simulink model "SynRM_Model_field"  (Simulink 7.9)
settings: Solver=ode3  StartTime=0.0  StopTime=1  FixedStep=.00001  RelTol=1e-3
undefined symbols (not defined in the file): I_s_max, J, K_iid, K_iiq, K_ipd, K_ipq, K_wd, K_wi, K_wp, L_d, L_q, P_r, r_s, Ts_id, Ts_iq, U_max
libraries: simulink x7, simulink_extras x1
settings Model: Creator=KHANSED  LastModifiedBy=KHANSED

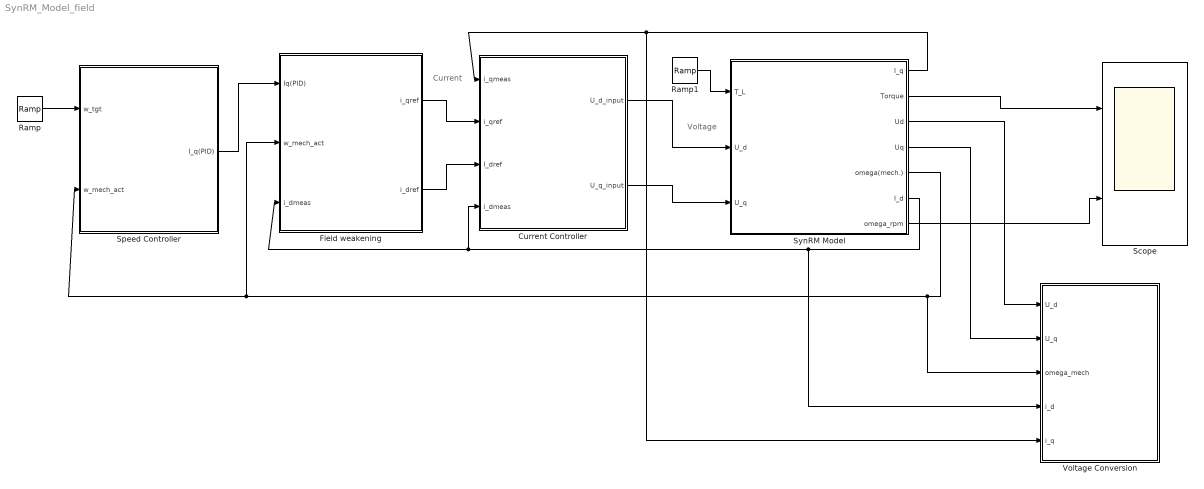
== system SynRM_Model_field ==
  note: Voltage
  note: Current
  Current Controller : Subsystem
  Field weakening : Subsystem
  Ramp : simulink/Sources/Ramp  slope=1500  start=0  X0=0
  Ramp1 : simulink/Sources/Ramp  slope=0  start=0.2  X0=0
  Scope : Scope  NumInputPorts=2
      settings: TimeRange=1  YMin=-0.012~-90.75  YMax=0.001~-89.7
  Speed Controller : Subsystem
  SynRM Model : Subsystem
  Voltage Conversion : Subsystem
  wires:
  SynRM Model/1(I_q) -> Current Controller/1(i_qmeas), Voltage Conversion/5(i_q)
  SynRM Model/6(I_d) -> Current Controller/4(i_dmeas), Field weakening/3(i_dmeas), Voltage Conversion/4(i_d)
  SynRM Model/5(omega(mech.)) -> Speed Controller/2(w_mech_act), Field weakening/2(w_mech_act), Voltage Conversion/3(omega_mech)
  Current Controller/1(U_d_input) -> SynRM Model/2(U_d)
  Current Controller/2(U_q_input) -> SynRM Model/3(U_q)
  SynRM Model/3(Ud) -> Voltage Conversion/1(U_d)
  SynRM Model/4(Uq) -> Voltage Conversion/2(U_q)
  SynRM Model/7(omega_rpm) -> Scope/2
  SynRM Model/2(Torque) -> Scope/1
  Ramp1/1 -> SynRM Model/1(T_L)
  Speed Controller/1(I_q(PID)) -> Field weakening/1(Iq(PID))
  Field weakening/2(i_dref) -> Current Controller/3(I_dref)
  Field weakening/1(i_qref) -> Current Controller/2(i_qref)
  Ramp/1 -> Speed Controller/1(w_tgt)

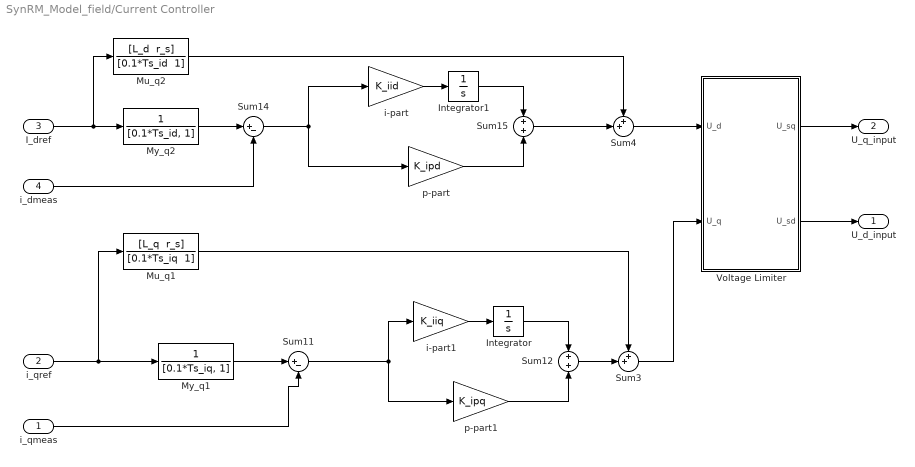
== system SynRM_Model_field/Current Controller ==
  i_qmeas : Inport
  i_qref : Inport  Port=2
  I_dref : Inport  Port=3
  i_dmeas : Inport  Port=4
  Integrator : Integrator
  Integrator1 : Integrator
  Mu_q1 : TransferFcn  Numerator="[L_q  r_s]"  Denominator="[0.1*Ts_iq  1]"
  Mu_q2 : TransferFcn  Numerator="[L_d  r_s]"  Denominator="[0.1*Ts_id  1]"
  My_q1 : TransferFcn  Denominator=[0.1*Ts_iq, 1]
  My_q2 : TransferFcn  Denominator=[0.1*Ts_id, 1]
  Sum11 : Sum  Inputs=|+-
  Sum12 : Sum
  Sum14 : Sum  Inputs=|+-
  Sum15 : Sum
  Sum3 : Sum  Inputs=++|
  Sum4 : Sum  Inputs=++|
  Voltage Limiter : Subsystem
  i-part : Gain  Gain=K_iid
  i-part1 : Gain  Gain=K_iiq
  p-part : Gain  Gain=K_ipd
  p-part1 : Gain  Gain=K_ipq
  U_d_input : Outport
  U_q_input : Outport  Port=2
  wires:
  p-part1/1 -> Sum12/2
  Integrator/1 -> Sum12/1
  i-part1/1 -> Integrator/1
  i_qmeas/1 -> Sum11/2
  p-part/1 -> Sum15/2
  Integrator1/1 -> Sum15/1
  i-part/1 -> Integrator1/1
  Sum11/1 -> i-part1/1, p-part1/1
  i_dmeas/1 -> Sum14/2
  Sum12/1 -> Sum3/2
  Sum15/1 -> Sum4/2
  Sum4/1 -> Voltage Limiter/1(U_d)
  Voltage Limiter/1(U_sq) -> U_q_input/1
  Voltage Limiter/2(U_sd) -> U_d_input/1
  My_q1/1 -> Sum11/1
  i_qref/1 -> My_q1/1, Mu_q1/1
  I_dref/1 -> My_q2/1, Mu_q2/1
  My_q2/1 -> Sum14/1
  Mu_q2/1 -> Sum4/1
  Mu_q1/1 -> Sum3/1
  Sum14/1 -> i-part/1, p-part/1
  Sum3/1 -> Voltage Limiter/2(U_q)

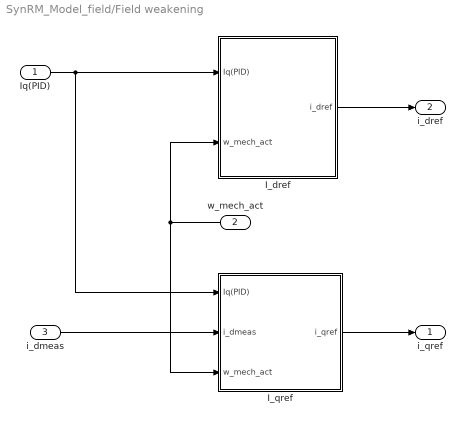
== system SynRM_Model_field/Field weakening ==
  Iq(PID) : Inport
  w_mech_act : Inport  Port=2
  i_dmeas : Inport  Port=3
  I_dref : Subsystem
  I_qref : Subsystem
  i_qref : Outport
  i_dref : Outport  Port=2
  wires:
  Iq(PID)/1 -> I_dref/1(Iq(PID)), I_qref/1(Iq(PID))
  w_mech_act/1 -> I_dref/2(w_mech_act), I_qref/3(w_mech_act)
  I_dref/1(i_dref) -> i_dref/1
  I_qref/1(i_qref) -> i_qref/1
  i_dmeas/1 -> I_qref/2(i_dmeas)

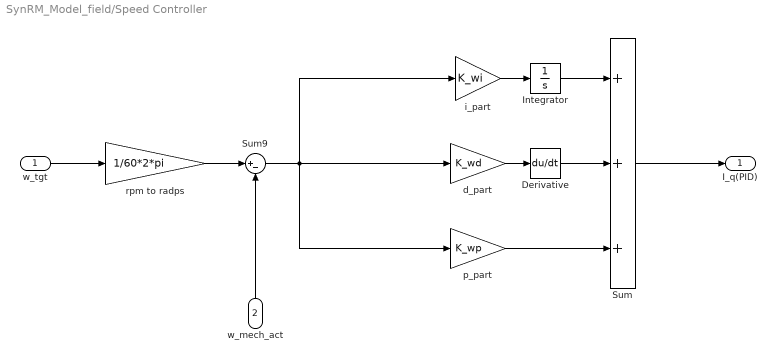
== system SynRM_Model_field/Speed Controller ==
  w_tgt : Inport
  w_mech_act : Inport  Port=2
  Derivative : Derivative
  Integrator : Integrator
  Sum : Sum  Inputs=+++
  Sum9 : Sum  Inputs=|+-
  d_part : Gain  Gain=K_wd
  i_part : Gain  Gain=K_wi
  p_part : Gain  Gain=K_wp
  rpm to radps : Gain  Gain=1/60*2*pi
  I_q(PID) : Outport
  wires:
  d_part/1 -> Derivative/1
  w_mech_act/1 -> Sum9/2
  Derivative/1 -> Sum/2
  p_part/1 -> Sum/3
  Sum9/1 -> p_part/1, d_part/1, i_part/1
  Integrator/1 -> Sum/1
  rpm to radps/1 -> Sum9/1
  w_tgt/1 -> rpm to radps/1
  i_part/1 -> Integrator/1
  Sum/1 -> I_q(PID)/1

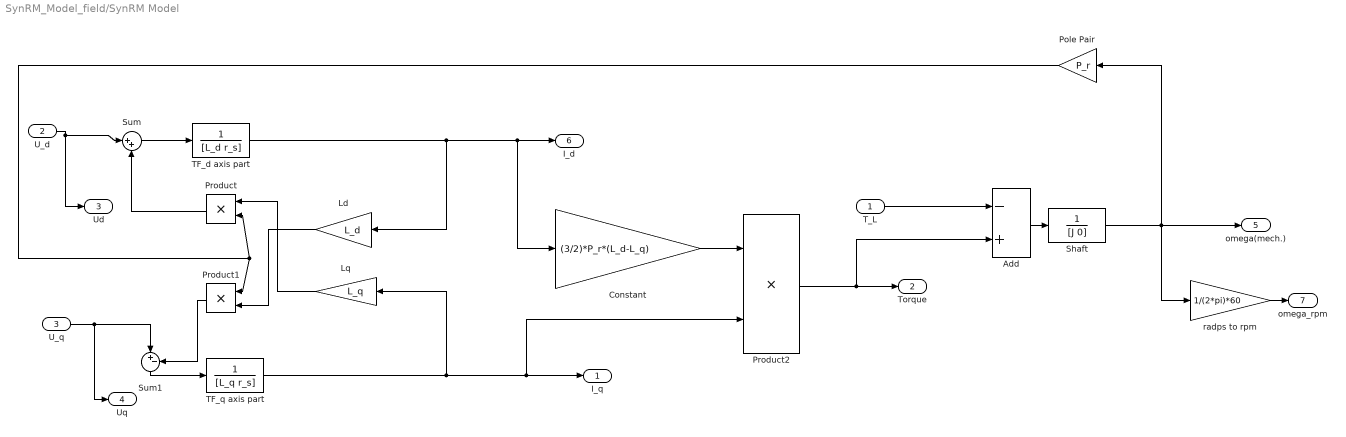
== system SynRM_Model_field/SynRM Model ==
  T_L : Inport
  U_d : Inport  Port=2
  U_q : Inport  Port=3
  Add : Sum  Inputs=-+
  Constant : Gain  Gain=(3/2)*P_r*(L_d-L_q)
  Ld : Gain  Gain=L_d
  Lq : Gain  Gain=L_q
  Pole Pair : Gain  Gain=P_r
  Product : Product  RndMeth=Zero
  Product1 : Product  RndMeth=Zero
  Product2 : Product  RndMeth=Zero
  Shaft : TransferFcn  Denominator=[J 0]
  Sum : Sum  Inputs=|++
  Sum1 : Sum  Inputs=|+-
  TF_d axis part : TransferFcn  Denominator=[L_d r_s]
  TF_q axis part : TransferFcn  Denominator=[L_q r_s]
  radps to rpm : Gain  Gain=1/(2*pi)*60
  I_q : Outport
  Torque : Outport  Port=2
  Ud : Outport  Port=3
  Uq : Outport  Port=4
  omega(mech.) : Outport  Port=5
  I_d : Outport  Port=6
  omega_rpm : Outport  Port=7
  wires:
  TF_d axis part/1 -> Ld/1, Constant/1, I_d/1
  Sum/1 -> TF_d axis part/1
  Lq/1 -> Product/1
  Ld/1 -> Product1/2
  TF_q axis part/1 -> Lq/1, Product2/2, I_q/1
  Product2/1 -> Torque/1, Add/2
  Constant/1 -> Product2/1
  Pole Pair/1 -> Product1/1, Product/2
  T_L/1 -> Add/1
  Sum1/1 -> TF_q axis part/1
  Product/1 -> Sum/2
  Product1/1 -> Sum1/2
  Add/1 -> Shaft/1
  Shaft/1 -> radps to rpm/1, Pole Pair/1, omega(mech.)/1
  U_d/1 -> Sum/1, Ud/1
  U_q/1 -> Sum1/1, Uq/1
  radps to rpm/1 -> omega_rpm/1

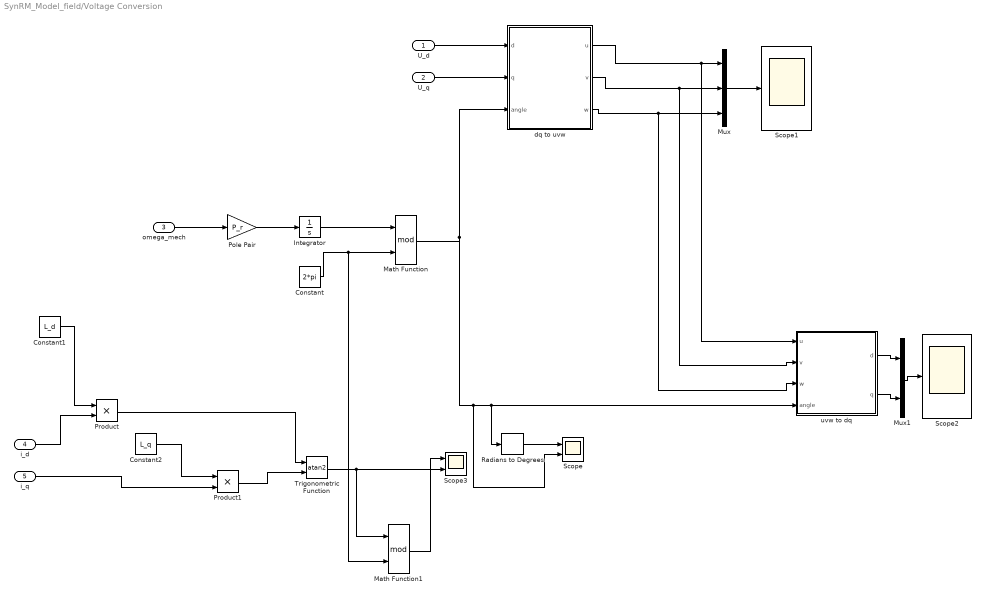
== system SynRM_Model_field/Voltage Conversion ==
  U_d : Inport
  U_q : Inport  Port=2
  omega_mech : Inport  Port=3
  i_d : Inport  Port=4
  i_q : Inport  Port=5
  Constant : Constant  Value=2*pi
  Constant1 : Constant  Value=L_d
  Constant2 : Constant  Value=L_q
  Integrator : Integrator
  Math Function : Math  Operator=mod  SaturateOnIntegerOverflow=on
  Math Function1 : Math  Operator=mod  SaturateOnIntegerOverflow=on
  Mux : Mux  Inputs=3
  Mux1 : Mux  Inputs=2
  Pole Pair : Gain  Gain=P_r
  Product : Product  RndMeth=Zero
  Product1 : Product  RndMeth=Zero
  Radians to Degrees : simulink_extras/Transformations/Radians to Degrees
  Scope : Scope  NumInputPorts=2
      settings: YMin=0~-5  YMax=375~5  SaveName=ScopeData6
  Scope1 : Scope
      settings: TimeRange=1  YMin=-1750  YMax=1750  SaveName=ScopeData3
  Scope2 : Scope
      settings: TimeRange=1  YMin=-250  YMax=25  SaveName=ScopeData7
  Scope3 : Scope  NumInputPorts=2
      settings: YMin=0.03~0.03  YMax=0.09~0.09
  Trigonometric Function : Trigonometry  Operator=atan2
  dq to uvw : Subsystem
  uvw to dq : Subsystem
  wires:
  dq to uvw/3(w) -> Mux/3, uvw to dq/3(w)
  Mux/1 -> Scope1/1
  Pole Pair/1 -> Integrator/1
  Constant/1 -> Math Function/2, Math Function1/2
  U_d/1 -> dq to uvw/1(d)
  U_q/1 -> dq to uvw/2(q)
  omega_mech/1 -> Pole Pair/1
  Integrator/1 -> Math Function/1
  dq to uvw/1(u) -> Mux/1, uvw to dq/1(u)
  dq to uvw/2(v) -> Mux/2, uvw to dq/2(v)
  Math Function/1 -> dq to uvw/3(angle), uvw to dq/4(angle), Radians to Degrees/1, Scope/2
  uvw to dq/1(d) -> Mux1/1
  uvw to dq/2(q) -> Mux1/2
  Mux1/1 -> Scope2/1
  Radians to Degrees/1 -> Scope/1
  i_d/1 -> Product/2
  i_q/1 -> Product1/2
  Product/1 -> Trigonometric Function/1
  Product1/1 -> Trigonometric Function/2
  Trigonometric Function/1 -> Scope3/2, Math Function1/1
  Math Function1/1 -> Scope3/1
  Constant1/1 -> Product/1
  Constant2/1 -> Product1/1

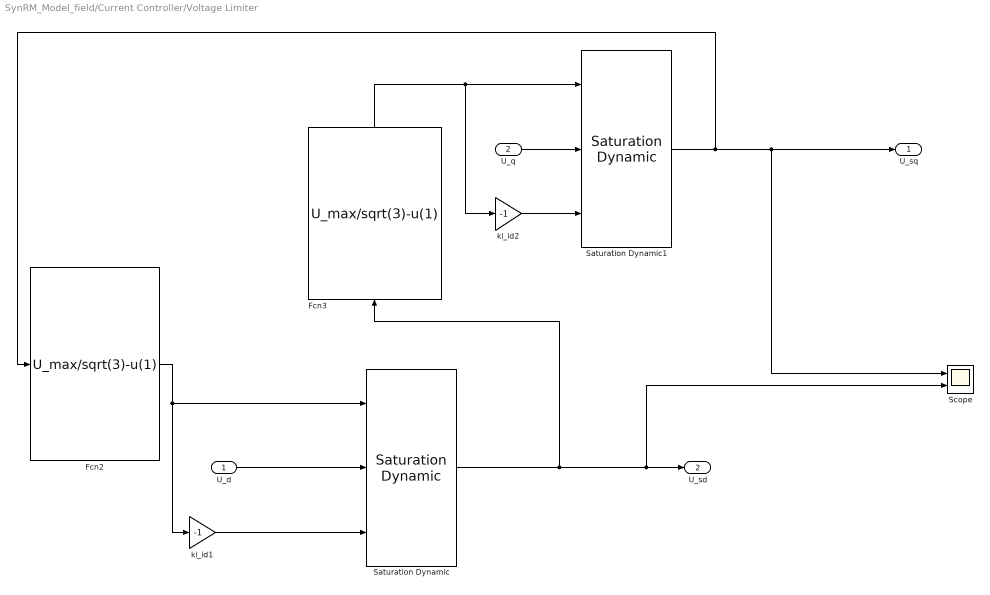
== system SynRM_Model_field/Current Controller/Voltage Limiter ==
  U_d : Inport
  U_q : Inport  Port=2
  Fcn2 : Fcn  Expr=U_max/sqrt(3)-u(1)
  Fcn3 : Fcn  Expr=U_max/sqrt(3)-u(1)
  Saturation Dynamic : simulink/Discontinuities/Saturation Dynamic  OutMin=[.001]  OutMax=[U_max]  OutDataTypeStr=Inherit: Same as second input  OutDataType=fixdt(1, 16)  OutScaling=2^-10  DoSatur=off
  Saturation Dynamic1 : simulink/Discontinuities/Saturation Dynamic  OutMin=[0.001]  OutMax=[U_max]  OutDataTypeStr=Inherit: Same as second input  OutDataType=fixdt(1, 16)  OutScaling=2^-10  DoSatur=off
  Scope : Scope  NumInputPorts=2
      settings: YMin=-5~-5  YMax=5~5  SaveName=ScopeData2
  ki_id1 : Gain  Gain=-1
  ki_id2 : Gain  Gain=-1
  U_sq : Outport
  U_sd : Outport  Port=2
  wires:
  ki_id1/1 -> Saturation Dynamic/3
  Saturation Dynamic/1 -> Fcn3/1, U_sd/1, Scope/2
  U_d/1 -> Saturation Dynamic/2
  Fcn2/1 -> Saturation Dynamic/1, ki_id1/1
  Saturation Dynamic1/1 -> Fcn2/1, U_sq/1, Scope/1
  U_q/1 -> Saturation Dynamic1/2
  Fcn3/1 -> Saturation Dynamic1/1, ki_id2/1
  ki_id2/1 -> Saturation Dynamic1/3

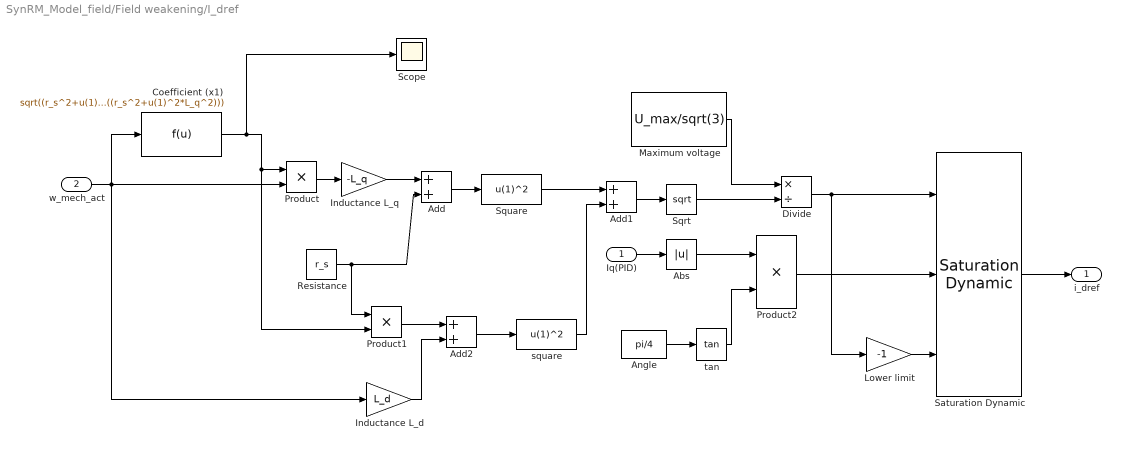
== system SynRM_Model_field/Field weakening/I_dref ==
  Iq(PID) : Inport
  w_mech_act : Inport  Port=2
  Abs : Abs
  Add : Sum
  Add1 : Sum
  Add2 : Sum
  Angle : Constant  Value=pi/4
  Coefficient (x1) : Fcn  Expr=sqrt((r_s^2+u(1)^2*L_d^2)/((r_s^2+u(1)^2*L_q^2)))
  Divide : Product  Inputs=*/
  Inductance L_d : Gain  Gain=L_d
  Inductance L_q : Gain  Gain=-L_q
  Lower limit : Gain  Gain=-1
  Maximum voltage : Constant  Value=U_max/sqrt(3)
  Product : Product  RndMeth=Zero
  Product1 : Product  RndMeth=Zero
  Product2 : Product  RndMeth=Zero
  Resistance : Constant  Value=r_s
  Saturation Dynamic : simulink/Discontinuities/Saturation Dynamic  OutMin=[]  OutMax=[]  OutDataTypeStr=Inherit: Same as second input  OutDataType=fixdt(1, 16)  OutScaling=2^-10  DoSatur=off
  Scope : Scope
      settings: SaveName=ScopeData5
  Sqrt : Sqrt  SaturateOnIntegerOverflow=on
  Square : Fcn  Expr=u(1)^2
  square : Fcn  Expr=u(1)^2
  "tan " : Trigonometry  Operator=tan
  i_dref : Outport
  wires:
  Product/1 -> Inductance L_q/1
  Inductance L_q/1 -> Add/1
  Resistance/1 -> Add/2, Product1/1
  Add/1 -> Square/1
  Square/1 -> Add1/1
  Product1/1 -> Add2/1
  Inductance L_d/1 -> Add2/2
  Add2/1 -> square/1
  square/1 -> Add1/2
  Add1/1 -> Sqrt/1
  Maximum voltage/1 -> Divide/1
  Sqrt/1 -> Divide/2
  "tan "/1 -> Product2/2
  Lower limit/1 -> Saturation Dynamic/3
  Divide/1 -> Lower limit/1, Saturation Dynamic/1
  Product2/1 -> Saturation Dynamic/2
  Coefficient (x1)/1 -> Product/1, Product1/2, Scope/1
  Angle/1 -> "tan "/1
  Saturation Dynamic/1 -> i_dref/1
  Iq(PID)/1 -> Abs/1
  Abs/1 -> Product2/1
  w_mech_act/1 -> Inductance L_d/1, Coefficient (x1)/1, Product/2

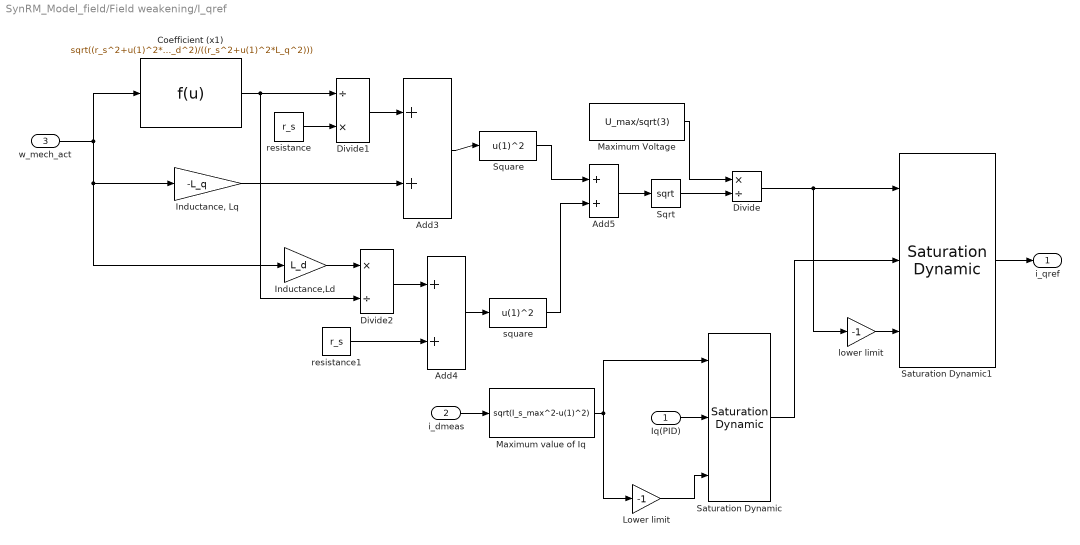
== system SynRM_Model_field/Field weakening/I_qref ==
  Iq(PID) : Inport
  i_dmeas : Inport  Port=2
  w_mech_act : Inport  Port=3
  Add3 : Sum
  Add4 : Sum
  Add5 : Sum
  Coefficient (x1) : Fcn  Expr=sqrt((r_s^2+u(1)^2*L_d^2)/((r_s^2+u(1)^2*L_q^2)))
  Divide : Product  Inputs=*/
  Divide1 : Product  Inputs=/*
  Divide2 : Product  Inputs=*/
  "Inductance, Lq" : Gain  Gain=-L_q
  Inductance,Ld : Gain  Gain=L_d
  Lower limit : Gain  Gain=-1
  Maximum Voltage : Constant  Value=U_max/sqrt(3)
  Maximum value of Iq : Fcn  Expr=sqrt(I_s_max^2-u(1)^2)
  Saturation Dynamic : simulink/Discontinuities/Saturation Dynamic  OutMin=[]  OutMax=[]  OutDataTypeStr=Inherit: Same as second input  OutDataType=fixdt(1, 16)  OutScaling=2^-10  DoSatur=off
  Saturation Dynamic1 : simulink/Discontinuities/Saturation Dynamic  OutMin=[]  OutMax=[]  OutDataTypeStr=Inherit: Same as second input  OutDataType=fixdt(1, 16)  OutScaling=2^-10  DoSatur=off
  Sqrt : Sqrt  SaturateOnIntegerOverflow=on
  Square : Fcn  Expr=u(1)^2
  lower limit : Gain  Gain=-1
  resistance : Constant  Value=r_s
  resistance1 : Constant  Value=r_s
  square : Fcn  Expr=u(1)^2
  i_qref : Outport
  wires:
  Maximum Voltage/1 -> Divide/1
  Coefficient (x1)/1 -> Divide2/2, Divide1/1
  Divide1/1 -> Add3/1
  "Inductance, Lq"/1 -> Add3/2
  Add3/1 -> Square/1
  Inductance,Ld/1 -> Divide2/1
  Divide2/1 -> Add4/1
  resistance1/1 -> Add4/2
  Add4/1 -> square/1
  Square/1 -> Add5/1
  square/1 -> Add5/2
  Add5/1 -> Sqrt/1
  Sqrt/1 -> Divide/2
  Iq(PID)/1 -> Saturation Dynamic/2
  lower limit/1 -> Saturation Dynamic1/3
  Divide/1 -> Saturation Dynamic1/1, lower limit/1
  Lower limit/1 -> Saturation Dynamic/3
  w_mech_act/1 -> Coefficient (x1)/1, "Inductance, Lq"/1, Inductance,Ld/1
  Saturation Dynamic/1 -> Saturation Dynamic1/2
  Saturation Dynamic1/1 -> i_qref/1
  i_dmeas/1 -> Maximum value of Iq/1
  Maximum value of Iq/1 -> Saturation Dynamic/1, Lower limit/1
  resistance/1 -> Divide1/2

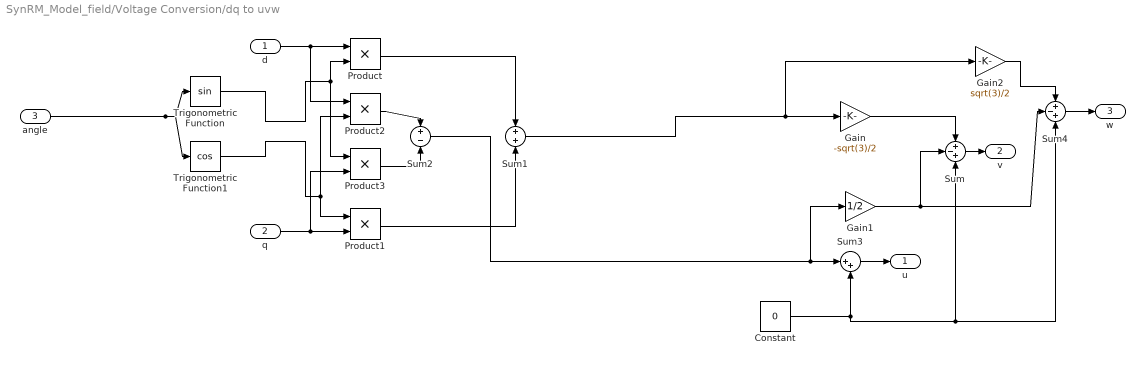
== system SynRM_Model_field/Voltage Conversion/dq to uvw ==
  d : Inport
  q : Inport  Port=2
  angle : Inport  Port=3
  Constant : Constant  Value=0
  Gain : Gain  Gain=-sqrt(3)/2
  Gain1 : Gain  Gain=1/2
  Gain2 : Gain  Gain=sqrt(3)/2
  Product{,1..3} (4 alike) : Product  RndMeth=Zero
  Sum : Sum  Inputs=+-+
  Sum1 : Sum  Inputs=+|+
  Sum2 : Sum  Inputs=+|-
  Sum3 : Sum  Inputs=|++
  Sum4 : Sum  Inputs=+-+
  Trigonometric Function : Trigonometry
  Trigonometric Function1 : Trigonometry  Operator=cos
  u : Outport
  v : Outport  Port=2
  w : Outport  Port=3
  wires:
  d/1 -> Product/1, Product2/1
  q/1 -> Product1/2, Product3/2
  Trigonometric Function/1 -> Product/2, Product3/1
  Trigonometric Function1/1 -> Product1/1, Product2/2
  Product/1 -> Sum1/1
  Product1/1 -> Sum1/2
  Product2/1 -> Sum2/1
  Product3/1 -> Sum2/2
  Sum2/1 -> Gain1/1, Sum3/1
  Sum4/1 -> w/1
  Sum/1 -> v/1
  Gain2/1 -> Sum4/1
  Gain1/1 -> Sum4/2, Sum/2
  Gain/1 -> Sum/1
  Sum3/1 -> u/1
  Constant/1 -> Sum4/3, Sum/3, Sum3/2
  angle/1 -> Trigonometric Function1/1, Trigonometric Function/1
  Sum1/1 -> Gain/1, Gain2/1

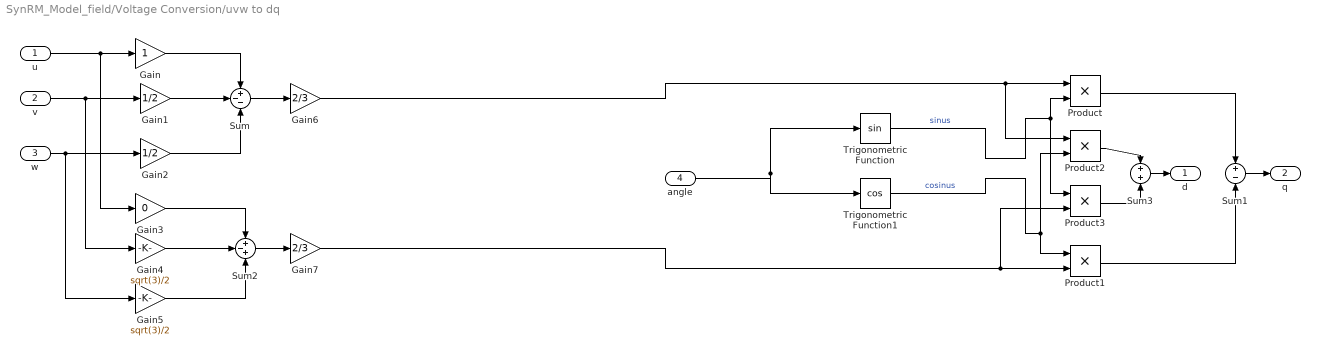
== system SynRM_Model_field/Voltage Conversion/uvw to dq ==
  u : Inport
  v : Inport  Port=2
  w : Inport  Port=3
  angle : Inport  Port=4
  Gain : Gain
  Gain1 : Gain  Gain=1/2
  Gain2 : Gain  Gain=1/2
  Gain3 : Gain  Gain=0
  Gain4 : Gain  Gain=sqrt(3)/2
  Gain5 : Gain  Gain=sqrt(3)/2
  Gain6 : Gain  Gain=2/3
  Gain7 : Gain  Gain=2/3
  Product{,1..3} (4 alike) : Product  RndMeth=Zero
  Sum : Sum  Inputs=+--
  Sum1 : Sum  Inputs=+|-
  Sum2 : Sum  Inputs=+-+
  Sum3 : Sum  Inputs=+|+
  Trigonometric Function : Trigonometry
  Trigonometric Function1 : Trigonometry  Operator=cos
  d : Outport
  q : Outport  Port=2
  wires:
  Gain/1 -> Sum/1
  Gain1/1 -> Sum/2
  Gain2/1 -> Sum/3
  Gain3/1 -> Sum2/1
  Gain4/1 -> Sum2/2
  Gain5/1 -> Sum2/3
  u/1 -> Gain/1, Gain3/1
  v/1 -> Gain1/1, Gain4/1
  w/1 -> Gain2/1, Gain5/1
  Sum/1 -> Gain6/1
  Sum2/1 -> Gain7/1
  Trigonometric Function/1 -> Product/2, Product3/1  "sinus"
  Trigonometric Function1/1 -> Product1/1, Product2/2  "cosinus"
  Product/1 -> Sum1/1
  Product1/1 -> Sum1/2
  Product2/1 -> Sum3/1
  Product3/1 -> Sum3/2
  Sum1/1 -> q/1
  Sum3/1 -> d/1
  angle/1 -> Trigonometric Function/1, Trigonometric Function1/1
  Gain6/1 -> Product/1, Product2/1
  Gain7/1 -> Product1/2, Product3/2
